simulink model "Double_inertia_integrator_method"  (R2024a)
settings: Solver=VariableStepAuto  StartTime=0.0  StopTime=10.0  RelTol=1e-3
values from neighbouring files (symbols this model uses):
  b1 = 1    [Second_order_parameters.mat]
  b2 = 50    [Second_order_parameters.mat]
  j1 = 100    [Second_order_parameters.mat]
  j2 = 10    [Second_order_parameters.mat]
  k1 = 4000    [Second_order_parameters.mat]
  k2 = 10    [Second_order_parameters.mat]
  k3 = 500    [Second_order_parameters.mat]
settings Model: Creator=nassa  LastModifiedBy=nassa

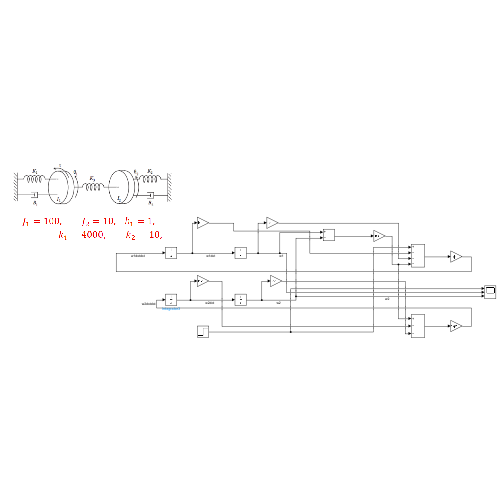
[thumbnail: Simulink's stored preview of the top-level diagram]
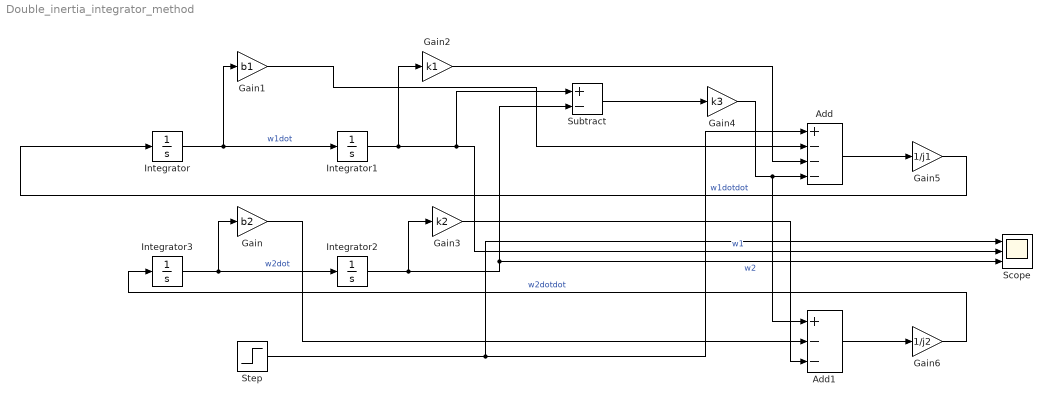
== system Double_inertia_integrator_method ==
  Add : Sum  Inputs=+---
  Add1 : Sum  Inputs=+--
  Gain : Gain  Gain=b2
  Gain1 : Gain  Gain=b1
  Gain2 : Gain  Gain=k1
  Gain3 : Gain  Gain=k2
  Gain4 : Gain  Gain=k3
  Gain5 : Gain  Gain=1/j1
  Gain6 : Gain  Gain=1/j2
  Integrator{,1..3} (4 alike) : Integrator
  Scope : Scope  NumInputPorts=3
  Step : Step  SampleTime=0
  Subtract : Sum  Inputs=+-
  wires:
  Integrator/1 -> Gain1/1, Integrator1/1  "w1dot"
  Integrator1/1 -> Scope/2, Subtract/1, Gain2/1  "w1"
  Gain5/1 -> Integrator/1  "w1dotdot"
  Integrator3/1 -> Gain/1, Integrator2/1  "w2dot"
  Integrator2/1 -> Scope/3, Subtract/2, Gain3/1  "w2"
  Gain6/1 -> Integrator3/1  "w2dotdot"
  Subtract/1 -> Gain4/1
  Step/1 -> Scope/1, Add/1
  Gain1/1 -> Add/2
  Gain2/1 -> Add/3
  Gain4/1 -> Add1/1, Add/4
  Add/1 -> Gain5/1
  Gain/1 -> Add1/2
  Gain3/1 -> Add1/3
  Add1/1 -> Gain6/1
